simulink model "FaultDataGeneratorNew"  (R2016b)
settings: Solver=ode15s  StartTime=0.0  StopTime=3500  MaxStep=0.001  RelTol=1e-3  EnableMultiTasking=on
values from neighbouring files (symbols this model uses):
  bigpump_const = 1    [run_model.m]
  fault_time = randi([200 1400])    [generate_training_data.m]
  minipump_const = 0    [run_model.m]
  time_const = 700    [run_model.m]
  ws_fault_time = fault_time    [run_model.m]
  ws_sample_time_end_valve_bigpump_in = 0    [run_model.m]
  ws_sample_time_end_valve_bigpump_out = 0    [run_model.m]
  ws_sample_time_end_valve_car_tank = 0    [run_model.m]
  ws_sample_time_end_valve_cartank1_in = 0    [run_model.m]
  ws_sample_time_end_valve_cartank1_out = 0    [run_model.m]
  ws_sample_time_end_valve_cartank2_in = 0    [run_model.m]
  ws_sample_time_end_valve_cartank2_out = 0    [run_model.m]
  ws_sample_time_end_valve_cartank3_in = 0    [run_model.m]
  ws_sample_time_end_valve_cartank3_out = 0    [run_model.m]
  ws_sample_time_end_valve_general_tank = 0    [run_model.m]
  ws_sample_time_end_valve_minipump_in = 0    [run_model.m]
  ws_sample_time_end_valve_minipump_out = 0    [run_model.m]
settings Model: Creator=Александр  LastModifiedBy=plotb
settings DataIOCC: LimitDataPoints=on
settings OptimizationCC: LifeSpan=inf
settings DebuggingCC: AllowSymbolicDim=off  SFUnexpectedBacktrackingDiag=warning  SFNoUnconditionalDefaultTransitionDiag=warning  SFExecutionAtInitializationDiag=none
settings ModelReferenceCC: PropagateSignalLabelsOutOfModel=off
settings GRTTargetCC: TargetLangStandard=C89/C90 (ANSI)
settings ConfigComp: CovMetricSettings=dw  CovHtmlReporting=on  CovSaveCumulativeToWorkspaceVar=on  CovSaveSingleToWorkspaceVar=on  CovExternalEMLEnable=off

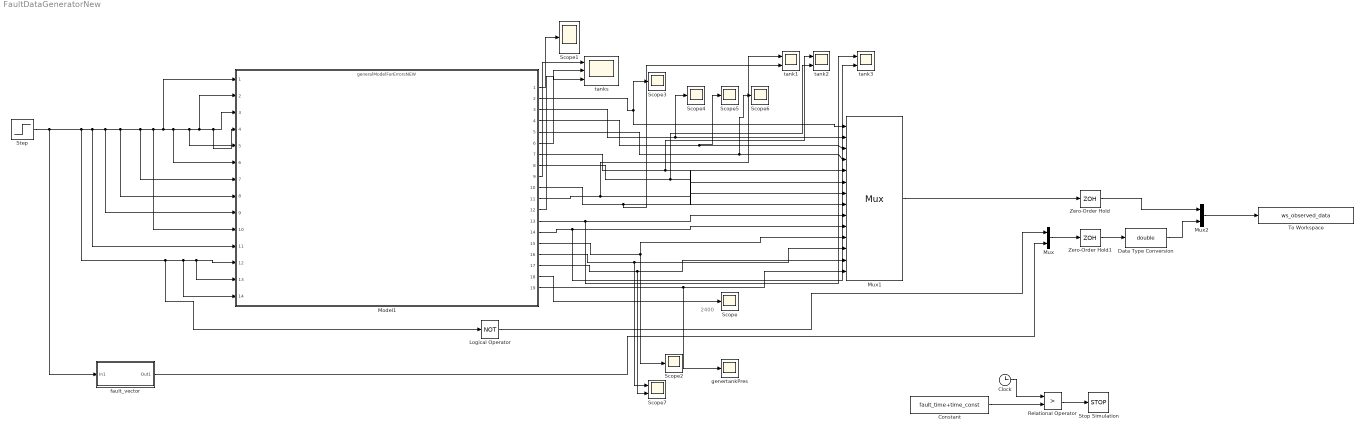
== system FaultDataGeneratorNew ==
  note: 2400
  Clock : Clock
  Constant : Constant  Value=fault_time+time_const
  Data Type Conversion : DataTypeConversion  OutDataTypeStr=double
  Logical Operator : Logic  Operator=NOT  AllPortsSameDT=off  OutDataTypeStr=boolean
  Model1 : ModelReference  ModelNameDialog=generalModelForErrorsNEW.slx  SimulationMode=Normal  ModelReferenceVersion=1.72
  Mux : Mux  Inputs=2
  Mux1 : Mux  Inputs=14
  Mux2 : Mux  Inputs=2
  Relational Operator : RelationalOperator  Operator=>  OutDataTypeStr=boolean  RndMeth=Simplest
  Scope{,1..6} (7 alike) : Scope
  Scope7 : Scope  NumInputPorts=2
  Step : Step  SampleTime=ws_fault_time
  Stop Simulation : Stop
  To Workspace : ToWorkspace  VariableName=ws_observed_data  SampleTime=0.1
  Zero-Order Hold : ZeroOrderHold  SampleTime=0.1
  Zero-Order Hold1 : ZeroOrderHold  SampleTime=0.1
  fault_vector : Subsystem
  genertankPres : Scope
  tank1 : Scope  NumInputPorts=2
  tank2 : Scope  NumInputPorts=2
  tank3 : Scope  NumInputPorts=2
  tanks : Scope  NumInputPorts=3
  wires:
  Model1/1 -> Scope1/1
  Model1/6 -> tanks/2
  Model1/12 -> tanks/3
  Model1/9 -> tanks/1
  Model1/18 -> Scope/1
  Step/1 -> fault_vector/1(In1), Logical Operator/1, Model1/14, Model1/13, Model1/12, Model1/11, Model1/9, Model1/8, Model1/7, Model1/10, Model1/1, Model1/6, Model1/5, Model1/2, Model1/4, Model1/3
  Model1/2 -> Mux1/1, Scope3/1
  Model1/3 -> Scope4/1, Mux1/2
  Model1/4 -> Scope5/1, Mux1/3
  Model1/5 -> Scope6/1, Mux1/4
  Model1/11 -> tank1/1, Mux1/5
  Model1/10 -> tank1/2, Mux1/6
  Model1/7 -> tank2/1, Mux1/7
  Model1/8 -> tank2/2, Mux1/8
  Model1/13 -> tank3/1, Mux1/9
  Model1/14 -> tank3/2, Mux1/10
  Model1/16 -> Scope7/1, Mux1/12
  Model1/17 -> Scope7/2, Mux1/13
  Model1/19 -> Mux1/14, genertankPres/1
  Zero-Order Hold/1 -> Mux2/1
  Clock/1 -> Relational Operator/1
  Constant/1 -> Relational Operator/2
  Relational Operator/1 -> Stop Simulation/1
  Model1/15 -> Scope2/1, Mux1/11
  Logical Operator/1 -> Mux/1
  fault_vector/1(Out1) -> Mux/2
  Mux1/1 -> Zero-Order Hold/1
  Mux/1 -> Zero-Order Hold1/1
  Mux2/1 -> To Workspace/1
  Zero-Order Hold1/1 -> Data Type Conversion/1
  Data Type Conversion/1 -> Mux2/2

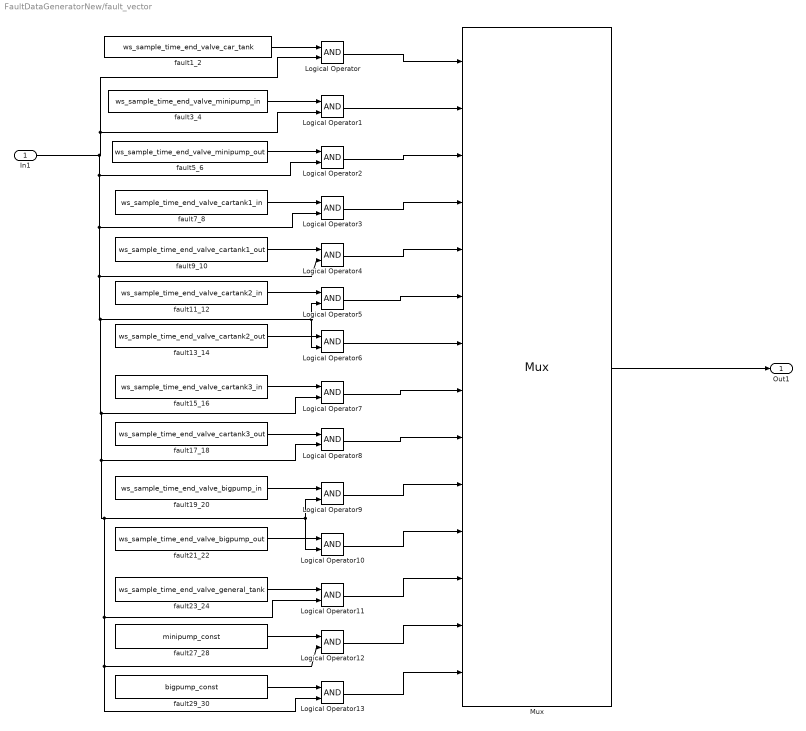
== system FaultDataGeneratorNew/fault_vector ==
  In1 : Inport
  Logical Operator{,1..13} (14 alike) : Logic  AllPortsSameDT=off  OutDataTypeStr=boolean
  Mux : Mux  Inputs=14
  fault11_12 : Constant  Value=ws_sample_time_end_valve_cartank2_in
  fault13_14 : Constant  Value=ws_sample_time_end_valve_cartank2_out
  fault15_16 : Constant  Value=ws_sample_time_end_valve_cartank3_in
  fault17_18 : Constant  Value=ws_sample_time_end_valve_cartank3_out
  fault19_20 : Constant  Value=ws_sample_time_end_valve_bigpump_in
  fault1_2 : Constant  Value=ws_sample_time_end_valve_car_tank
  fault21_22 : Constant  Value=ws_sample_time_end_valve_bigpump_out
  fault23_24 : Constant  Value=ws_sample_time_end_valve_general_tank
  fault27_28 : Constant  Value=minipump_const
  fault29_30 : Constant  Value=bigpump_const
  fault3_4 : Constant  Value=ws_sample_time_end_valve_minipump_in
  fault5_6 : Constant  Value=ws_sample_time_end_valve_minipump_out
  fault7_8 : Constant  Value=ws_sample_time_end_valve_cartank1_in
  fault9_10 : Constant  Value=ws_sample_time_end_valve_cartank1_out
  Out1 : Outport
  wires:
  fault1_2/1 -> Logical Operator/1
  In1/1 -> Logical Operator13/2, Logical Operator12/2, Logical Operator11/2, Logical Operator10/2, Logical Operator9/2, Logical Operator8/2, Logical Operator7/2, Logical Operator6/2, Logical Operator5/2, Logical Operator4/2, Logical Operator3/2, Logical Operator2/2, Logical Operator1/2, Logical Operator/2
  Mux/1 -> Out1/1
  fault3_4/1 -> Logical Operator1/1
  fault5_6/1 -> Logical Operator2/1
  fault7_8/1 -> Logical Operator3/1
  fault9_10/1 -> Logical Operator4/1
  fault11_12/1 -> Logical Operator5/1
  fault17_18/1 -> Logical Operator8/1
  fault15_16/1 -> Logical Operator7/1
  fault13_14/1 -> Logical Operator6/1
  fault19_20/1 -> Logical Operator9/1
  fault21_22/1 -> Logical Operator10/1
  fault23_24/1 -> Logical Operator11/1
  fault27_28/1 -> Logical Operator12/1
  fault29_30/1 -> Logical Operator13/1
  Logical Operator/1 -> Mux/1
  Logical Operator1/1 -> Mux/2
  Logical Operator2/1 -> Mux/3
  Logical Operator3/1 -> Mux/4
  Logical Operator4/1 -> Mux/5
  Logical Operator5/1 -> Mux/6
  Logical Operator6/1 -> Mux/7
  Logical Operator7/1 -> Mux/8
  Logical Operator8/1 -> Mux/9
  Logical Operator9/1 -> Mux/10
  Logical Operator10/1 -> Mux/11
  Logical Operator11/1 -> Mux/12
  Logical Operator12/1 -> Mux/13
  Logical Operator13/1 -> Mux/14
